simulink library "NullCommandBus"  (R2018b)
settings: Solver=VariableStepAuto  StartTime=0.0  StopTime=10.0  RelTol=1e-3
settings Model: Creator=RA24876  LastModifiedBy=RA24876
settings SFSimCC: SimUseLocalCustomCode=off
settings RTWCC: RTWUseLocalCustomCode=off
settings CodeAppCC: StateflowObjectComments=on

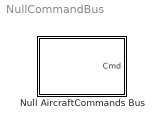
== system NullCommandBus ==
  Null AircraftCommands Bus : Subsystem  mask(Null AircraftCommands Bus){}
      mask help: Creates an AircraftCommands bus signal with all null values. Assign values to elements with a Bus Assignment block.

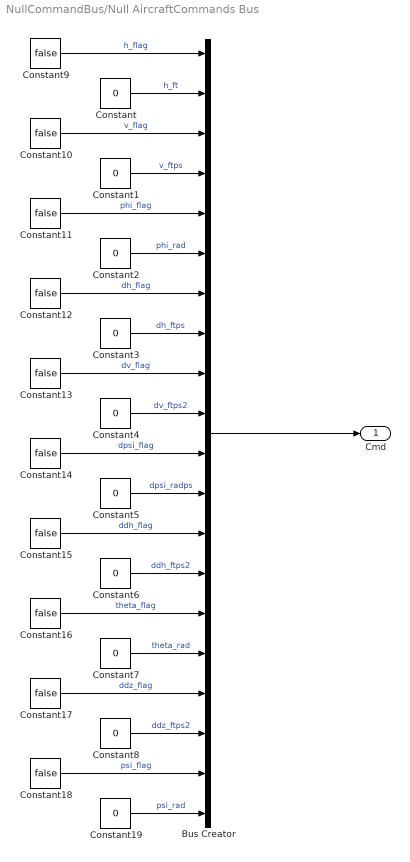
== system NullCommandBus/Null AircraftCommands Bus ==
  Bus Creator : BusCreator  Inputs=20  OutDataTypeStr=Bus: AircraftCommands
      settings: InheritFromInputs=off
  Constant{,1..8,19} (10 alike) : Constant  Value=0
  Constant{9..18} (10 alike) : Constant  Value=false  OutDataTypeStr=boolean
  Cmd : Outport  OutDataTypeStr=Bus: AircraftCommands
  wires:
  Bus Creator/1 -> Cmd/1
  Constant/1 -> Bus Creator/2  "h_ft"
  Constant1/1 -> Bus Creator/4  "v_ftps"
  Constant2/1 -> Bus Creator/6  "phi_rad"
  Constant3/1 -> Bus Creator/8  "dh_ftps"
  Constant4/1 -> Bus Creator/10  "dv_ftps2"
  Constant5/1 -> Bus Creator/12  "dpsi_radps"
  Constant6/1 -> Bus Creator/14  "ddh_ftps2"
  Constant7/1 -> Bus Creator/16  "theta_rad"
  Constant8/1 -> Bus Creator/18  "ddz_ftps2"
  Constant9/1 -> Bus Creator/1  "h_flag"
  Constant10/1 -> Bus Creator/3  "v_flag"
  Constant11/1 -> Bus Creator/5  "phi_flag"
  Constant12/1 -> Bus Creator/7  "dh_flag"
  Constant13/1 -> Bus Creator/9  "dv_flag"
  Constant14/1 -> Bus Creator/11  "dpsi_flag"
  Constant15/1 -> Bus Creator/13  "ddh_flag"
  Constant16/1 -> Bus Creator/15  "theta_flag"
  Constant17/1 -> Bus Creator/17  "ddz_flag"
  Constant19/1 -> Bus Creator/20  "psi_rad"
  Constant18/1 -> Bus Creator/19  "psi_flag"
